simulink model "modello_completo_simulink2019"  (R2019b)
settings: Solver=VariableStepAuto  StartTime=0.0  StopTime=10  RelTol=1e-3
values from neighbouring files (symbols this model uses):
  a = 0.35    [data.m]    (also in geodetic2nedS.m = 6378137)
  a1 = rho * D^4 * alpha1    (= 0.000388302366464)    [data.m]
  a2 = -rho * D^3 * alpha2 * (1 - omega)    (= 0.0037030698432)    [data.m]
  AHRS_bias = [0 0 0]    [data.m]
  AHRS_sample_time = 1/50    (= 0.02)    [data.m]
  AHRS_var = ([1 1 2] * pi/180).^2    [data.m]
  alpha1 = 0.0113    [data.m]
  alpha2 = -0.0091    [data.m]
  c = son2(1)    [Sonar_id.m]    (also in data.m = 0.19)
  current = [seaCurrent; 0; 0; 0]    [data.m]
  D = 0.076    [data.m]
  dead_zone_limit = 31.5    [data.m]
  DVL_sample_t = 1/12    (= 0.0833333333333)    [data.m]
  DVL_var1 = 0.005^2    (= 2.5e-05)    [data.m]
  DVL_var2 = 0.015^2    (= 0.000225)    [data.m]
  DVL_var3 = 0.023^2    (= 0.000529)    [data.m]
  gps_sample_t = 1    [data.m]
  H = eye(3)    [data.m]    (also in navigation_data.m)
  IMU_sample_time = 1/100    (= 0.01)    [data.m]
  initial = []    [data.m]
  INSP = unicode2native(inspectionDirection)    [data.m]
  Ki_bodypos1 = 0    [parametri_PID.m]
  Ki_bodypos2 = 0    [parametri_PID.m]
  Ki_bodypos3 = 0    [parametri_PID.m]
  Ki_bodypos4 = 0    [parametri_PID.m]
  Ki_bodypos5 = 0    [parametri_PID.m]
  Ki_depth1 = 0    [parametri_PID.m]
  Ki_depth2 = 0    [parametri_PID.m]
  Ki_depth3 = 0    [parametri_PID.m]
  Ki_depth4 = 0    [parametri_PID.m]
  Ki_depth5 = 0    [parametri_PID.m]
  Ki_latvel1 = 0    [parametri_PID.m]
  Ki_latvel2 = 0    [parametri_PID.m]
  Ki_latvel3 = 0    [parametri_PID.m]
  Ki_latvel4 = 0    [parametri_PID.m]
  Ki_latvel5 = 0    [parametri_PID.m]
  Ki_P1 = 0    [parametri_PID.m]
  Ki_P2 = 0    [parametri_PID.m]
  Ki_P3 = 0    [parametri_PID.m]
  Ki_P4 = 0    [parametri_PID.m]
  Ki_P5 = 0    [parametri_PID.m]
  Ki_R1 = 0    [parametri_PID.m]
  Ki_R2 = 0    [parametri_PID.m]
  Ki_R3 = 0    [parametri_PID.m]
  Ki_R4 = 0    [parametri_PID.m]
  Ki_R5 = 0    [parametri_PID.m]
  Ki_rel_or1 = 0    [parametri_PID.m]
  Ki_rel_or2 = 0    [parametri_PID.m]
  Ki_rel_or3 = 0    [parametri_PID.m]
  Ki_rel_or4 = 0    [parametri_PID.m]
  Ki_rel_or5 = 0    [parametri_PID.m]
  Ki_reldist1 = 0    [parametri_PID.m]
  Ki_reldist2 = 0    [parametri_PID.m]
  Ki_reldist3 = 0    [parametri_PID.m]
  Ki_reldist4 = 0    [parametri_PID.m]
  Ki_reldist5 = 0    [parametri_PID.m]
  Ki_surge1 = 0    [parametri_PID.m]
  Ki_surge2 = 0    [parametri_PID.m]
  Ki_surge3 = 0    [parametri_PID.m]
  Ki_surge4 = 0    [parametri_PID.m]
  Ki_surge5 = 0    [parametri_PID.m]
  Ki_yaw1 = 0    [parametri_PID.m]
  Ki_yaw2 = 0    [parametri_PID.m]
  Ki_yaw3 = 0    [parametri_PID.m]
  Ki_yaw4 = 0    [parametri_PID.m]
  Ki_yaw5 = 0    [parametri_PID.m]
  Kp_bodypos1 = 0    [parametri_PID.m]
  Kp_bodypos2 = 2    [parametri_PID.m]
  Kp_bodypos3 = 2    [parametri_PID.m]
  Kp_bodypos4 = 2    [parametri_PID.m]
  Kp_bodypos5 = 2    [parametri_PID.m]
  Kp_depth1 = 0    [parametri_PID.m]
  Kp_depth2 = 2    [parametri_PID.m]
  Kp_depth3 = 2    [parametri_PID.m]
  Kp_depth4 = 2    [parametri_PID.m]
  Kp_depth5 = 2    [parametri_PID.m]
  Kp_latvel1 = 0    [parametri_PID.m]
  Kp_latvel2 = 2    [parametri_PID.m]
  Kp_latvel3 = 2    [parametri_PID.m]
  Kp_latvel4 = 2    [parametri_PID.m]
  Kp_latvel5 = 2    [parametri_PID.m]
  Kp_P1 = 0    [parametri_PID.m]
  Kp_P2 = 2    [parametri_PID.m]
  Kp_P3 = 2    [parametri_PID.m]
  Kp_P4 = 2    [parametri_PID.m]
  Kp_P5 = 2    [parametri_PID.m]
  Kp_R1 = 0    [parametri_PID.m]
  Kp_R2 = 2    [parametri_PID.m]
  Kp_R3 = 2    [parametri_PID.m]
  Kp_R4 = 2    [parametri_PID.m]
  Kp_R5 = 2    [parametri_PID.m]
  Kp_rel_or1 = 0    [parametri_PID.m]
  Kp_rel_or2 = 2    [parametri_PID.m]
  Kp_rel_or3 = 2    [parametri_PID.m]
  Kp_rel_or4 = 2    [parametri_PID.m]
  Kp_rel_or5 = 2    [parametri_PID.m]
  Kp_reldist1 = 0    [parametri_PID.m]
  Kp_reldist2 = 2    [parametri_PID.m]
  Kp_reldist3 = 2    [parametri_PID.m]
  Kp_reldist4 = 2    [parametri_PID.m]
  Kp_reldist5 = 2    [parametri_PID.m]
  Kp_surge1 = 0    [parametri_PID.m]
  Kp_surge2 = 2    [parametri_PID.m]
  Kp_surge3 = 2    [parametri_PID.m]
  Kp_surge4 = 2    [parametri_PID.m]
  Kp_surge5 = 2    [parametri_PID.m]
  Kp_yaw1 = 0.6*6    (= 3.6)    [parametri_PID.m]
  Kp_yaw2 = 2    [parametri_PID.m]
  Kp_yaw3 = 2    [parametri_PID.m]
  Kp_yaw4 = 2    [parametri_PID.m]
  Kp_yaw5 = 2    [parametri_PID.m]
  M = M_rb + M_a    [Masse.m]
  M_inv = inv(M)    [Masse.m]
  n_max = 340    [data.m]
  num_cycle = 5    [data.m]    (also in navigation_data.m)
  omega = 0.1    [data.m]
  plot_smpl = 0.1    [data.m]
  ps_sample_t = 0.02    [data.m]
  ps_var = (5000/3)^2    (= 2777777.77778)    [data.m]
  pylonCenter = [ 43.723046 ... (first row only)    [missionB.m]
  ... (+4 more)
undefined symbols (not defined in the file or in its folder): DiscIntNeverNeededParam, s_data
libraries: simulink x3
(part 5 of 6)

== system modello_completo_simulink2019/Vehicle Model/Thrusters/T/Thruster 4 ==
  note: n is the rotational speed of the thruster
      | V is the speed component of the water along the thruster axis
      |
      | n is saturated according to data
      | a dead zone is considered according to data
      | the thruster is characterised by 1st order dynamics (tau = 0.2s)
  n [rad/s] : Inport
  V [m/s] : Inport  Port=2
  Dead Zone : DeadZone  LowerValue=-dead_zone_limit  UpperValue=dead_zone_limit  SaturateOnIntegerOverflow=on
  MATLAB Function : MATLAB Function  TreatAsAtomicUnit=on
  Saturation : Saturate  UpperLimit=n_max  LowerLimit=-n_max
  Transfer Fcn : TransferFcn  Denominator=[0.2 1]
  T i : Outport
  wires:
  V [m/s]/1 -> MATLAB Function/2(V)
  Saturation/1 -> MATLAB Function/1(n)
  Transfer Fcn/1 -> Saturation/1
  Dead Zone/1 -> Transfer Fcn/1
  n [rad/s]/1 -> Dead Zone/1
  MATLAB Function/1(T) -> T i/1

== system modello_completo_simulink2019/Vehicle Model/Thrusters/T/Thruster 5 ==
  note: n is the rotational speed of the thruster
      | V is the speed component of the water along the thruster axis
      |
      | n is saturated according to data
      | a dead zone is considered according to data
      | the thruster is characterised by 1st order dynamics (tau = 0.2s)
  n [rad/s] : Inport
  V [m/s] : Inport  Port=2
  Dead Zone : DeadZone  LowerValue=-dead_zone_limit  UpperValue=dead_zone_limit  SaturateOnIntegerOverflow=on
  MATLAB Function : MATLAB Function  TreatAsAtomicUnit=on
  Saturation : Saturate  UpperLimit=n_max  LowerLimit=-n_max
  Transfer Fcn : TransferFcn  Denominator=[0.2 1]
  T i : Outport
  wires:
  V [m/s]/1 -> MATLAB Function/2(V)
  Saturation/1 -> MATLAB Function/1(n)
  Transfer Fcn/1 -> Saturation/1
  Dead Zone/1 -> Transfer Fcn/1
  n [rad/s]/1 -> Dead Zone/1
  MATLAB Function/1(T) -> T i/1

== system modello_completo_simulink2019/Vehicle Model/Thrusters/T/Thruster 6 ==
  note: n is the rotational speed of the thruster
      | V is the speed component of the water along the thruster axis
      |
      | n is saturated according to data
      | a dead zone is considered according to data
      | the thruster is characterised by 1st order dynamics (tau = 0.2s)
  n [rad/s] : Inport
  V [m/s] : Inport  Port=2
  Dead Zone : DeadZone  LowerValue=-dead_zone_limit  UpperValue=dead_zone_limit  SaturateOnIntegerOverflow=on
  MATLAB Function : MATLAB Function  TreatAsAtomicUnit=on
  Saturation : Saturate  UpperLimit=n_max  LowerLimit=-n_max
  Transfer Fcn : TransferFcn  Denominator=[0.2 1]
  T i : Outport
  wires:
  V [m/s]/1 -> MATLAB Function/2(V)
  Saturation/1 -> MATLAB Function/1(n)
  Transfer Fcn/1 -> Saturation/1
  Dead Zone/1 -> Transfer Fcn/1
  n [rad/s]/1 -> Dead Zone/1
  MATLAB Function/1(T) -> T i/1

== system modello_completo_simulink2019/Vehicle Model/Thrusters/T/Thruster 7 ==
  note: n is the rotational speed of the thruster
      | V is the speed component of the water along the thruster axis
      |
      | n is saturated according to data
      | a dead zone is considered according to data
      | the thruster is characterised by 1st order dynamics (tau = 0.2s)
  n [rad/s] : Inport
  V [m/s] : Inport  Port=2
  Dead Zone : DeadZone  LowerValue=-dead_zone_limit  UpperValue=dead_zone_limit  SaturateOnIntegerOverflow=on
  MATLAB Function : MATLAB Function  TreatAsAtomicUnit=on
  Saturation : Saturate  UpperLimit=n_max  LowerLimit=-n_max
  Transfer Fcn : TransferFcn  Denominator=[0.2 1]
  T i : Outport
  wires:
  V [m/s]/1 -> MATLAB Function/2(V)
  Saturation/1 -> MATLAB Function/1(n)
  Transfer Fcn/1 -> Saturation/1
  Dead Zone/1 -> Transfer Fcn/1
  n [rad/s]/1 -> Dead Zone/1
  MATLAB Function/1(T) -> T i/1

== matlab function modello_completo_simulink2019/Vehicle Model/Model Vehicle/D ==
  data: ni_r input; F_d output; rho input
function F_d = D_forces(ni_r, rho)
    % Funzione per il calcolo delle forze di drag (Formulazione tratta da
    % Fossen(2011))
    %
    % IN: ni_r [6x1] | velocità lineare [3x1] m/s, velocità angolare [3x1] rad/s 
    %                  differenza tra velocità del centro di massa del
    %                  veicolo in terna NED e velocità della corrente
    %     rho  [1x1] | densità dell'acqua kg/m^3
    %
    % OUT: F_d [6x1] | forze [3x1] N, momenti [3x1] N*m dovuti a effetti di
    %                  drag
    %
    
    ni_lin = ni_r(1:3); 
    ni_ang = ni_r(4:6);
    
    % semiassi del veicolo
    a = 0.35; 
    b = a;
    c = 0.19;
    
    A_ab = pi*a*b;      % Area su cui agisce la forza di drag lin lungo z, momento di drag intorno a x e y
    A_bc = pi*b*c;      % Area su cui agisce la forza di drag lin lungo x, momento di drag intorno a z
    A_ac = pi*a*c;      % Area su cui agisce la forza di drag lin lungo y

    Di = 0.7; % diametro m massimo del veicolo, supposto il veicolo una sfera
    
    % Calcolo del numero di Reynolds basato su una velocità operativa di
    % 0.3 m/s, viscosità del fluido di 1e-3 Pa*s, calcolata a una
    % temperatura di 20 °C e con una densità di 1030 kg/m^3
    visc = 1e-3;
    vmax = 3e-1;
    rho  = 1030;
    Re = Di/(visc/rho)*vmax; % Re = 2*1e5
 
    Cd = 0.49; % Coefficiente di drag ricavato da Re nel caso di una sfera liscia
    
    % Calcolo dei raggi medi delle semiellisse di applicazione del momento
    % di drag
    
    rm_z = 4*c/(3*pi);
    rm_xy = 4*a/(3*pi);
    
    D_lin = -1/2*rho*Cd*diag([A_bc, A_ac, A_ab])*(abs(ni_lin).*ni_lin); % Forze lineari
    D_ang = -1/2*rho*Cd*diag([rm_xy^3*A_ab, rm_xy^3*A_ab, rm_z^3*A_bc])*(abs(ni_ang).*ni_ang); % Momenti
    
    F_d = [D_lin; D_ang];
end

== matlab function modello_completo_simulink2019/Vehicle Model/Model Vehicle/C ==
  data: ni_r input; F_c output; M input
function F_c = C(ni_r, M)
    % Funzione per il calcolo delle forze e dei momenti di Coriolis e
    % centripete (Formulazione tratta dal Fossen(2011))
    
    % IN: ni_r [6x1] | velocità lineare [3x1] m/s, velocità angolare [3x1] rad/s 
    %                  differenza tra velocità del centro di massa del
    %                  veicolo in terna NED e velocità della corrente
    %     M    [6x6] | matrice delle masse
    
    % OUT: F_c [6x1] | forze [3x1] N, momenti [3x1] N*m dovuti a effetti di
    %                  Coriolis e accelerazione centripeta
    
    ni = ni_r;
    M11 = M(1:3,1:3);
    M22 = M(4:6,4:6);
    ni1 = ni(1:3);
    ni2 = ni(4:6);
    C11 = zeros(3,3);
    s1 = M11*ni1;
    C12 = - [0 -s1(3) s1(2); s1(3) 0 -s1(1); -s1(2) s1(1) 0];
    C21 = C12;
    s2 = M22*ni2;
    C22 = - [0 -s2(3) s2(2); s2(3) 0 -s2(1); -s2(2) s2(1) 0];
    F_c = [C11 C12; C21 C22]*ni_r;
end

== matlab function modello_completo_simulink2019/Vehicle Model/Model Vehicle/grav ==
  data: rho input; eta input; F_g output
function F_g = grav(rho, eta)
    % Funzione per il calcolo delle forze di gravità e galleggiamento del
    % veicolo (Formulazione tratta da Fossen(2011))
    %
    % IN: rho  [1x1] | densità dell'acqua kg/m^3
    %     eta  [6x1] | posizione [3x1] m, orientazione [3x1] rad del veicolo in terna NED
    %
    % OUT: F_g [6x1] | forze [3x1] N, momenti [3x1] N*m dovuti a effetti di
    %                  gravità e galleggiamento
    %
    
    eta2 = eta(4:6);
    g = 9.81; % m/s^2 modulo della accelerazione di gravità
    
    % semiassi m del veicolo
    a = 0.35;
    b = a;
    c = 0.19;
    
    massa = 100; % massa kg del veicolo
    
    % Calcolo della calotta dell'ellissoide emersa dall'acqua per simulare 
    % il comportamento del veicolo emerso 
    
    if eta(3) >= c
       V = 4/3*pi*a*b*c; % volume del veicolo totalmente immerso
    else
       V = 4/3*pi*a*b*c - (pi*a*b/(3*c^2))*((eta(3)-c)^2)*(3*c - abs(eta(3) - c)); % volume del veicolo parzialmente immerso
    end
    
    
    W = massa*g; % modulo forza di gravità
    B = rho*V*g; % modulo forza di galleggiamento
    
    % Passaggio da terna NED a Body
    J = Jac(eta2);
    J1 = J(1:3,1:3);
    J2 = J(4:6,4:6);
    
    f_g = inv(J1)*[0; 0; W];
    f_b = inv(J1)*[0; 0; -B];
    r_g = [0; 0; 0]; % posizione del centro di massa
    r_b = [0; 0; -c/2]; % posizione del centro di galleggiamento

    F_g = -[f_g + f_b; cross(r_g,f_g) + cross(r_b,f_b)];
end

== matlab function modello_completo_simulink2019/Vehicle Model/Model Vehicle/Kinematic/Jac ==
  data: eta input; J output
function J = Jac(eta)
    % Funzione per il calcolo dello Jacobiano per il passaggio da
    % coordinate Body a coordinate NED
    %
    % IN: eta2 [3x1] rad angoli di roll, pitch, yaw
    %
    % OUT: J [6x6] Jacobiano complessivo
    %
    eta2 = eta(4:6);
    phi = eta2(1);
    theta = eta2(2);
    psi = eta2(3);
    Rx = [1 0 0; 0 cos(phi) sin(phi); 0 -sin(phi) cos(phi)]; % Rot elementare attorno a x
    Ry = [cos(theta) 0 -sin(theta); 0 1 0; sin(theta) 0 cos(theta)]; % Rot elementare attorno a y
    Rz = [cos(psi) sin(psi) 0; -sin(psi) cos(psi) 0; 0 0 1]; % Rot elementare attorno a z
    J1 = Rz'*Ry'*Rx'; % Jacobiano per il passaggio da Body a NED delle componenti lineari
    J2 = [1 sin(phi)*tan(theta) cos(phi)*tan(theta); ... % Jacobiano per il passaggio da Body a NED delle componenti angolari
        0 cos(phi) -sin(phi); ...
        0 sin(phi)/cos(theta) cos(phi)/cos(theta)];
    J = blkdiag(J1, J2);
end

== matlab function modello_completo_simulink2019/Vehicle Model/Thrusters/T/Thruster 1/MATLAB Function ==
  data: n input; T output; V input; D parameter; omega parameter; a1 parameter; a2 parameter; alpha1 parameter; alpha2 parameter
function T = thrusterModel(n, V, D, omega, a1, a2, alpha1, alpha2)

Va = (1-omega) * V;     % Advancement velocity at the propeller
J0 = Va/(n*D);          % Advancement Coefficient

if J0 > -alpha1/alpha2  % Out of linearity domain (right side)
    T = 0;              % A null generated thrust is assumed
    
elseif J0 < 0           % Out of linearity domain (left side)
    T = a1*abs(n)*n;    % Bollard thrust is assumed

else                    % Within the linearity domain
    T = a1*abs(n)*n - a2*abs(n)*V;
end

== matlab function modello_completo_simulink2019/Vehicle Model/Thrusters/T/Thruster 2/MATLAB Function ==
  data: n input; T output; V input; D parameter; omega parameter; a1 parameter; a2 parameter; alpha1 parameter; alpha2 parameter
function T = thrusterModel(n, V, D, omega, a1, a2, alpha1, alpha2)

Va = (1-omega) * V;     % Advancement velocity at the propeller
J0 = Va/(n*D);          % Advancement Coefficient

if J0 > -alpha1/alpha2  % Out of linearity domain (right side)
    T = 0;              % A null generated thrust is assumed
    
elseif J0 < 0           % Out of linearity domain (left side)
    T = a1*abs(n)*n;    % Bollard thrust is assumed

else                    % Within the linearity domain
    T = a1*abs(n)*n - a2*abs(n)*V;
end

== matlab function modello_completo_simulink2019/Vehicle Model/Thrusters/T/Thruster 3/MATLAB Function ==
  data: n input; T output; V input; D parameter; omega parameter; a1 parameter; a2 parameter; alpha1 parameter; alpha2 parameter
function T = thrusterModel(n, V, D, omega, a1, a2, alpha1, alpha2)

Va = (1-omega) * V;     % Advancement velocity at the propeller
J0 = Va/(n*D);          % Advancement Coefficient

if J0 > -alpha1/alpha2  % Out of linearity domain (right side)
    T = 0;              % A null generated thrust is assumed
    
elseif J0 < 0           % Out of linearity domain (left side)
    T = a1*abs(n)*n;    % Bollard thrust is assumed

else                    % Within the linearity domain
    T = a1*abs(n)*n - a2*abs(n)*V;
end

== matlab function modello_completo_simulink2019/Vehicle Model/Thrusters/T/Thruster 4/MATLAB Function ==
  data: n input; T output; V input; D parameter; omega parameter; a1 parameter; a2 parameter; alpha1 parameter; alpha2 parameter
function T = thrusterModel(n, V, D, omega, a1, a2, alpha1, alpha2)

Va = (1-omega) * V;     % Advancement velocity at the propeller
J0 = Va/(n*D);          % Advancement Coefficient

if J0 > -alpha1/alpha2  % Out of linearity domain (right side)
    T = 0;              % A null generated thrust is assumed
    
elseif J0 < 0           % Out of linearity domain (left side)
    T = a1*abs(n)*n;    % Bollard thrust is assumed

else                    % Within the linearity domain
    T = a1*abs(n)*n - a2*abs(n)*V;
end

== matlab function modello_completo_simulink2019/Vehicle Model/Thrusters/T/Thruster 5/MATLAB Function ==
  data: n input; T output; V input; D parameter; omega parameter; a1 parameter; a2 parameter; alpha1 parameter; alpha2 parameter
function T = thrusterModel(n, V, D, omega, a1, a2, alpha1, alpha2)

Va = (1-omega) * V;     % Advancement velocity at the propeller
J0 = Va/(n*D);          % Advancement Coefficient

if J0 > -alpha1/alpha2  % Out of linearity domain (right side)
    T = 0;              % A null generated thrust is assumed
    
elseif J0 < 0           % Out of linearity domain (left side)
    T = a1*abs(n)*n;    % Bollard thrust is assumed

else                    % Within the linearity domain
    T = a1*abs(n)*n - a2*abs(n)*V;
end

== matlab function modello_completo_simulink2019/Vehicle Model/Thrusters/T/Thruster 6/MATLAB Function ==
  data: n input; T output; V input; D parameter; omega parameter; a1 parameter; a2 parameter; alpha1 parameter; alpha2 parameter
function T = thrusterModel(n, V, D, omega, a1, a2, alpha1, alpha2)

Va = (1-omega) * V;     % Advancement velocity at the propeller
J0 = Va/(n*D);          % Advancement Coefficient

if J0 > -alpha1/alpha2  % Out of linearity domain (right side)
    T = 0;              % A null generated thrust is assumed
    
elseif J0 < 0           % Out of linearity domain (left side)
    T = a1*abs(n)*n;    % Bollard thrust is assumed

else                    % Within the linearity domain
    T = a1*abs(n)*n - a2*abs(n)*V;
end

== matlab function modello_completo_simulink2019/Vehicle Model/Thrusters/T/Thruster 7/MATLAB Function ==
  data: n input; T output; V input; D parameter; omega parameter; a1 parameter; a2 parameter; alpha1 parameter; alpha2 parameter
function T = thrusterModel(n, V, D, omega, a1, a2, alpha1, alpha2)

Va = (1-omega) * V;     % Advancement velocity at the propeller
J0 = Va/(n*D);          % Advancement Coefficient

if J0 > -alpha1/alpha2  % Out of linearity domain (right side)
    T = 0;              % A null generated thrust is assumed
    
elseif J0 < 0           % Out of linearity domain (left side)
    T = a1*abs(n)*n;    % Bollard thrust is assumed

else                    % Within the linearity domain
    T = a1*abs(n)*n - a2*abs(n)*V;
end

== matlab function modello_completo_simulink2019/Vehicle Model/Model Vehicle/MATLAB Function ==
  data: coord_pylon input; eta input; eta_ecef output
function eta_ecef = nedToEcef(coord_pylon, eta) 
    % Funzione per il passaggio da coordinate in terna NED a coordinate in
    % terna geodetica.
    %
    % IN: coord_pylon [3x1] | latitudine e longitudine [2x1] deg,
    %                         profondità [1x1] m
    %     eta         [6x1] | posizione [3x1] m, orientazione [3x1] rad 
    %                         del veicolo in terna NED
    
    % OUT: eta_ecef   [6x1] | posizione [3x1] m, orientazione [3x1] rad 
    %                         del veicolo in terna ecef
    
    coder.extrinsic('wgs84Ellipsoid');

    coder.extrinsic('ned2geodetic');
    
    eta_pos = eta(1:6);
    wgs84 = wgs84Ellipsoid('meter'); 
    [eta_pos(1), eta_pos(2)] = ned2geodetic(eta(1), eta(2), eta(3), coord_pylon(1), coord_pylon(2), coord_pylon(3), wgs84, 'degrees');
    
    eta_pos(3) = eta(3);
    eta_pos(4:6) = eta_pos(4:6);
    
    eta_ecef = eta_pos;
    
end

== matlab function modello_completo_simulink2019/Vehicle Model/MATLAB Function ==
  data: eta input; ni_c output; current input
function ni_c = current_ned2body(eta, current)
    % Funzione per il calcolo della velocità della corrente in terna Body
    
    % IN: eta     [6x1] | posizione [3x1] m, orientazione [3x1] rad del veicolo in terna NED
    %     current [6x1] | velocità lineare [3x1] m/s, velocità angolare
    %                     [3x1] rad/s (sempre nulla) della corrente in
    %                     terna NED


    % OUT: ni_c   [6x1] | velocità lineare [3x1] m/s, velocità angolare
    %                     [3x1] rad/s (sempre nulla) della corrente in
    %                     terna Body
    
    eta2 = eta(4:6);            % eta2 espresso in radianti
    ni_c = Jac(eta2)'*current;
end

== matlab function modello_completo_simulink2019/Vehicle Model/Thrusters/T/MATLAB Function ==
  data: ni_r input; v_th output
function v_th = thrusters(ni_r) 
    % Funzione per valutare le componenti di velocità di ciascun thruster
    % in direzione del proprio asse 
    
    % IN: ni_r [6x1] | velocità lineare [3x1] m/s, velocità angolare [3x1] rad/s 
    %                  differenza tra velocità del centro di massa del
    %                  veicolo in terna NED e velocità della corrente

    
    % OUT: v_th [7x1] m/s componenti di velocità relativa lungo l'asse di
    % ciascun thruster
    
    % posizionamento dei thrusters
    p1 = [0 -0.25 0]';
    p2 = [0 0.25 0]';
    p3 = [-0.25 0 0]';
    p4 = [0.25 0 0]';
    p5 = [-0.15 -0.15 0]';
    p6 = [-0.15 0.15 0]';
    p7 = [0.15 0 0]';


    % versori posizionamento dei thrusters
    t1 = [1 0 0]';
    t2 = t1;
    t3 = [0 1 0]';
    t4 = -t3;
    t5 = [0 0 1]';
    t6 = t5;
    t7 = t5;

    v_lin = ni_r(1:3); % componenti di velocità lineare
    v_ang = ni_r(4:6); % componenti di velocità angolare

    % velocità lineari dei punti p_i (centro dei thrusters) attraverso la formula
    % fondamentale della cinematica
    vp1 = v_lin + cross(v_ang, p1); 
    vp2 = v_lin + cross(v_ang, p2);
    vp3 = v_lin + cross(v_ang, p3);
    vp4 = v_lin + cross(v_ang, p4);
    vp5 = v_lin + cross(v_ang, p5);
    vp6 = v_lin + cross(v_ang, p6);
    vp7 = v_lin + cross(v_ang, p7);

    % velocità relativa lungo l'asse di ciascun thruster 
    v1 = vp1'*t1;
    v2 = vp2'*t2;
    v3 = vp3'*t3;
    v4 = vp4'*t4;
    v5 = vp5'*t5;
    v6 = vp6'*t6;
    v7 = vp7'*t7;

    v_th = [ v1 v2 v3 v4 v5 v6 v7]'; % OUT
end

== matlab function modello_completo_simulink2019/Navigation1/Geodetic to NED/MATLAB Function2 ==
  data: GPS_geodetic input; GPS_flag input; GPS_NED output; depth input; pylonCenter parameter
function GPS_NED = Geo2NED(GPS_geodetic, GPS_flag, depth, pylonCenter)

% Funzione che trasforma le coordinate dal sistema di riferimento geodetico
% ad un sistema NED con origine in corrispondenza del centro del pilone.

%% GPS non funzionante
if GPS_flag == 0            
    GPS_NED = [0;0;0];
    return
end

%% Variabili
phi = GPS_geodetic(1);                  % Coordinate geodetiche in radianti                     
lambda = GPS_geodetic(2);  
h = -depth;

phi_pyl = pylonCenter(1) * pi/180;      % Origine del sistema NED in coordinate geodetiche
lambda_pyl = pylonCenter(2) * pi/180;

%% Trasformazione coordinate
coder.extrinsic('wgs84Ellipsoid');
coder.extrinsic('geodetic2ned');
    
[x_gps2, y_gps2, z_gps2] = geodetic2ned(phi, lambda, -depth, phi_pyl, lambda_pyl, 0, wgs84Ellipsoid, 'radians');
eta_NED_GPS = [x_gps2; y_gps2];

GPS_NED = zeros(3,1);
GPS_NED(1) = eta_NED_GPS(1);            % Coordiante NED in radianti
GPS_NED(2) = eta_NED_GPS(2);
GPS_NED(3) = GPS_flag;

== matlab function modello_completo_simulink2019/Vehicle Model/Thrusters/saturation_tau ==
  data: tau input; tau_sat output; eta input
function tau_sat = sat_tau(tau, eta)
    % Funzione per la saturazione della spinta verso l'alto in uscita al blocco 
    % dei thrusters nell'ipotesi in cui il veicolo si trovi in superficie
    % con angoli di yaw, pitch e roll supposti piccoli a piacere

    % IN: tau [6x1] | forze [3x1] N, momenti [3x1] N*m agenti sul veicolo
    %     eta [6x1] | posizione [3x1] m, orientazione [3x1] rad del veicolo in terna NED
    
    % OUT: tau_sat [6x1] | forze saturate [3x1] N e momenti [3x1] N*m agenti sul veicolo
    
    tau_sat = [0;0;0;0;0;0];
    tau_sat = tau;

    if eta(3) < 0.1 % condizione per il veicolo in superficie
        tau_sat(3) = 0;
    end
    
end

== matlab function modello_completo_simulink2019/Vehicle Model/MATLAB Function1 ==
  data: Tdes input; n output
function n  = fcn(Tdes)
n=zeros(1,7)';
a1=0.000388302366464000;
%assunzione modello a bassa velocità
for i=1:1:7
       n(i)=sign(Tdes(i))*sqrt((abs(Tdes(i))/a1));  
end
end

== matlab function modello_completo_simulink2019/Navigation1/MATLAB Function1 ==
  data: ang_vel input; DVL input; nu_1 output; c parameter
function nu_1  = dvl2body(ang_vel, DVL, c)

% Funzione che si occupa di trasformare la velocità da sistema di
% riferimento associato al DVL al sistema BODY

% nu_dvl = R_b^dvl (nu_1 + S(nu_2)* P_dvl)
% nu_1 = R_b^dvl' * nu_dvl - S(nu_2) * P_dvl

nu_1    =   zeros(4,1);
nu_2    =   [ang_vel(1); ang_vel(2); ang_vel(3)];
vel_dvl =   [DVL(1); DVL(2); DVL(3)];
R_b_dvl =   eye(3);

S = [   0,          -nu_2(3),   nu_2(2); 
        nu_2(3),    0,          -nu_2(1); 
        -nu_2(2),   nu_2(1),    0       ];
    
p = [0;0;c];

nu_1(1:3) = R_b_dvl' * vel_dvl - S * p;
nu_1(4) = DVL(4); %Flag

== matlab function modello_completo_simulink2019/Navigation1/MATLAB Function2 ==
  data: Depth_ps input; Depth output; c parameter
function  Depth = ps2body(Depth_ps, c)
% Il profondimetro è posizionato nella parte inferiore dell'AUV, lungo
% l'asse z
Depth = zeros(2,1);
Depth(1) = Depth_ps(1) - c;     %profondità rispetto al centro di massa
Depth(2) = Depth_ps(2);         %flag

== matlab function modello_completo_simulink2019/Navigation1/AHRS_function ==
  data: eta2 output; lin_acc input; nu2 output; ang_vel input; orientation input
function [eta2, nu2]= AHRS_signals(lin_acc, ang_vel, orientation)
acc = lin_acc(1:3);
nu2 = ang_vel(1:3);
eta2 = orientation(1:3);

== matlab function modello_completo_simulink2019/Navigation1/DVL_function ==
  data: dvl input; velocity_est output; flag_DVL output
function [velocity_est, flag_DVL] = DVL_signals(dvl)
velocity_est = dvl(1:3);
flag_DVL = dvl(4);

== matlab function modello_completo_simulink2019/Navigation1/NED to Geodetic/MATLAB Function1 ==
  data: eta_NED input; eta_geodetic output; depth input; pylonCenter parameter
function eta_geodetic = NED2Geo(eta_NED, depth, pylonCenter)

% Funzione che trasforma le coordinate dal sistema NED con origine in
% corrispondenza del centro del pilone al sistema di riferimento geodetico

phi_pyl = pylonCenter(1) * pi/180;      % Origine del sistema NED in coordinate geodetiche 
lambda_pyl = pylonCenter(2) * pi/180;

%% Trasformazione
coder.extrinsic('wgs84Ellipsoid');
coder.extrinsic('ned2geodetic');

[lat, lon, h] = ned2geodetic(eta_NED(1), eta_NED(2), depth, phi_pyl, lambda_pyl, 0, wgs84Ellipsoid, 'radians');

eta_geodetic = [0; 0];
eta_geodetic = [lat; lon];              % Coordiante geodetiche in radianti

== matlab function modello_completo_simulink2019/Navigation1/Relative estimation/Sonar trigger/MATLAB Function ==
  data: sonar input; sum input; pulse output; prev output
function [pulse, prev] = fcn(sonar, sum)

% La funzione si occupa di monitorare la misura dei sonar,
% quando esse sono modificate manda un impulso al blocco di stima relativa

if nnz(isnan(sum)) > 0 || nnz(sum) == 0 
    pulse = 0;
else
    pulse = 1;
end

prev = sonar;

== matlab function modello_completo_simulink2019/Navigation1/Relative estimation/Subsystem/MATLAB Function9 ==
  data: sonar input; orientation input; distance output; alpha output; flag_sonar output; pylonRadius parameter; a parameter; s_data parameter
function [distance, alpha, flag_sonar] = relative_values(sonar, orientation, pylonRadius, a, s_data)

% Chiamando la funzione "fcn_sonar" si occupa di calcolate la distanza
% e l'angolo dell'AUV rispetto al pilone

distance = 0;
alpha = 0;
flag_sonar = 0;

coder.extrinsic('fcn_sonar');

[distance, alpha, flag_sonar] = fcn_sonar(sonar, orientation, pylonRadius, a, s_data);
end

== matlab function modello_completo_simulink2019/Navigation1/flag_function ==
  data: flag_depth input; flag_AHRS input; error_flag output; flag_DVL input; flag_sonar input
function error_flag = fcn(flag_depth, flag_AHRS, flag_DVL, flag_sonar)

% Funzione che rileva la presenza di errore in un sensore

flag_ahrs = flag_AHRS(1) & flag_AHRS(2) & flag_AHRS(3);
error_flag = ~(flag_depth & flag_ahrs & flag_DVL & flag_sonar); % Vale 1 se vi è un errore

== matlab function modello_completo_simulink2019/Navigation1/z_EKF/EXTENDED KALMAN FILTER/Correzione  ==
  data: prev_pos output; prev_pos input; P input; hat input; meas_pos input; GPS_flag input; meas_depth input; P output; hat output; R parameter; H parameter
function [prev_pos, P, hat] = EKF_pos(prev_pos, P, hat, meas_pos, GPS_flag, meas_depth, R, H)
%% EKF: Correction

% Il filtro corregge i valori di posizione x e y solo quando è disponibile una nuova misura del GPS
if nnz(round(10.^4*(meas_pos - prev_pos))/10.^4) ~= 0 && GPS_flag == 1       % Se il flag è 0 il GPS non funziona

    z_tilde = [ meas_pos(1) - hat(1);
                meas_pos(2) - hat(2);
                meas_depth - hat(3)];

else
        z_tilde = [ 0;
                    0;
                meas_depth - hat(3)];
end
            
    S = H * P * H' + R;

    K = P * H' * S^(-1);
    
    hat = hat + K * z_tilde;
    P = (eye(3) - K * H) * P;  

prev_pos = meas_pos;

== matlab function modello_completo_simulink2019/Navigation1/z_EKF/EXTENDED KALMAN FILTER/Predizione ==
  data: P input; hat input; dT input; P output; hat output; orientation input; dvl input; ahrs_flag input; init input; P0 input; Q parameter
function [P, hat]  = EKF_pos(P, hat, dT, orientation, dvl, ahrs_flag, init, P0, Q)

dvl_flag = dvl(4);

%% Inizializzazione stato e matrice P
if nnz(hat) == 0           
    hat= init;
    P = P0;
end

if (ahrs_flag && dvl_flag) == 1
    %% Calcolo variabili e matrici
    phi     =   orientation(1);             % roll
    theta   =   orientation(2);             % pitch
    psi_    =   orientation(3);             % yaw
    vel     =   [dvl(1); dvl(2); dvl(3)];  
    
    J       =   zeros(3,3);
    Lk      =   zeros(3,6);
    
    J = [ cos(psi_)*cos(theta), cos(psi_)*sin(phi)*sin(theta) - cos(phi)*sin(psi_), sin(phi)*sin(psi_) + cos(phi)*cos(psi_)*sin(theta);
       cos(theta)*sin(psi_), cos(phi)*cos(psi_) + sin(phi)*sin(psi_)*sin(theta), cos(phi)*sin(psi_)*sin(theta) - cos(psi_)*sin(phi);
         -sin(theta),                                cos(theta)*sin(phi),                                cos(phi)*cos(theta)];
     
    x = dvl(1);
    y = dvl(2);
    z = dvl(3);
    n_ahrs1 = 0;
    n_ahrs2 = 0;
    n_ahrs3 = 0;

    % Matrice Lk: derivata della funzione f rispetto al rumore di AHRS e
    % DVL
    Lk = [  dT*(y*(sin(n_ahrs1 + phi)*sin(n_ahrs3 + psi_) + cos(n_ahrs1 + phi)*cos(n_ahrs3 + psi_)*sin(n_ahrs2 + theta)) + z*(cos(n_ahrs1 + phi)*sin(n_ahrs3 + psi_) - cos(n_ahrs3 + psi_)*sin(n_ahrs1 + phi)*sin(n_ahrs2 + theta))), dT*(z*cos(n_ahrs1 + phi)*cos(n_ahrs3 + psi_)*cos(n_ahrs2 + theta) - x*cos(n_ahrs3 + psi_)*sin(n_ahrs2 + theta) + y*cos(n_ahrs3 + psi_)*cos(n_ahrs2 + theta)*sin(n_ahrs1 + phi)), -dT*(y*(cos(n_ahrs1 + phi)*cos(n_ahrs3 + psi_) + sin(n_ahrs1 + phi)*sin(n_ahrs3 + psi_)*sin(n_ahrs2 + theta)) - z*(cos(n_ahrs3 + psi_)*sin(n_ahrs1 + phi) - cos(n_ahrs1 + phi)*sin(n_ahrs3 + psi_)*sin(n_ahrs2 + theta)) + x*cos(n_ahrs2 + theta)*sin(n_ahrs3 + psi_)), dT*cos(n_ahrs3 + psi_)*cos(n_ahrs2 + theta), -dT*(cos(n_ahrs1 + phi)*sin(n_ahrs3 + psi_) - cos(n_ahrs3 + psi_)*sin(n_ahrs1 + phi)*sin(n_ahrs2 + theta)),  dT*(sin(n_ahrs1 + phi)*sin(n_ahrs3 + psi_) + cos(n_ahrs1 + phi)*cos(n_ahrs3 + psi_)*sin(n_ahrs2 + theta));
     -dT*(y*(cos(n_ahrs3 + psi_)*sin(n_ahrs1 + phi) - cos(n_ahrs1 + phi)*sin(n_ahrs3 + psi_)*sin(n_ahrs2 + theta)) + z*(cos(n_ahrs1 + phi)*cos(n_ahrs3 + psi_) + sin(n_ahrs1 + phi)*sin(n_ahrs3 + psi_)*sin(n_ahrs2 + theta))), dT*(z*cos(n_ahrs1 + phi)*cos(n_ahrs2 + theta)*sin(n_ahrs3 + psi_) - x*sin(n_ahrs3 + psi_)*sin(n_ahrs2 + theta) + y*cos(n_ahrs2 + theta)*sin(n_ahrs1 + phi)*sin(n_ahrs3 + psi_)),  dT*(z*(sin(n_ahrs1 + phi)*sin(n_ahrs3 + psi_) + cos(n_ahrs1 + phi)*cos(n_ahrs3 + psi_)*sin(n_ahrs2 + theta)) - y*(cos(n_ahrs1 + phi)*sin(n_ahrs3 + psi_) - cos(n_ahrs3 + psi_)*sin(n_ahrs1 + phi)*sin(n_ahrs2 + theta)) + x*cos(n_ahrs3 + psi_)*cos(n_ahrs2 + theta)), dT*cos(n_ahrs2 + theta)*sin(n_ahrs3 + psi_),  dT*(cos(n_ahrs1 + phi)*cos(n_ahrs3 + psi_) + sin(n_ahrs1 + phi)*sin(n_ahrs3 + psi_)*sin(n_ahrs2 + theta)), -dT*(cos(n_ahrs3 + psi_)*sin(n_ahrs1 + phi) - cos(n_ahrs1 + phi)*sin(n_ahrs3 + psi_)*sin(n_ahrs2 + theta));
                                                                                                                                    dT*(y*cos(n_ahrs1 + phi)*cos(n_ahrs2 + theta) - z*cos(n_ahrs2 + theta)*sin(n_ahrs1 + phi)),                                                            -dT*(x*cos(n_ahrs2 + theta) + z*cos(n_ahrs1 + phi)*sin(n_ahrs2 + theta) + y*sin(n_ahrs1 + phi)*sin(n_ahrs2 + theta)),                                                                                                                                                                                                                                                                      0,                    -dT*sin(n_ahrs2 + theta),                                                                 dT*cos(n_ahrs2 + theta)*sin(n_ahrs1 + phi),                                                                 dT*cos(n_ahrs1 + phi)*cos(n_ahrs2 + theta)];

    %% EKF: Predizione

    hat  =  hat + dT * J * vel;        
    P =  P + Lk * Q * Lk';            

 
end

== matlab function modello_completo_simulink2019/Navigation1/z_EKF/Trigger & Init/Depth trigger/MATLAB Function ==
  data: count input; count output; dT output; depth input; sum input; pulse output; prev output
function [count, dT, pulse, prev] = fcn(count, depth, sum)

% La funzione si occupa di monitorare la misura del profondimetro,
% quando essa è modificata manda un impulso al blocco EKF e il tempo
% trascorso dalla precedente variazione

dT = 0;  

if nnz(round(10.^4*sum )/10.^4) == 0
    pulse = 0;
    count = count + 1;
else
    pulse = 1;
    dT = count * (1/200);
    count = 1;
end

prev = depth;

== matlab function modello_completo_simulink2019/Env. & Sensor Model1/AHRS SENSOR/    ==
  data: ni_1 input; ni_1_dot input; lin_acc output; ang_vel output; m output; ni_2 input; eta_2 input; eta_2_dot input
function [lin_acc, ang_vel, m] = IMU(ni_1, ni_1_dot, ni_2, eta_2, eta_2_dot)

% questa funzione, partendo dalle informazioni cinematiche dell' AUV
% restituisce in output delle misure di accelerazione, velocità angolare
% e campo magnetico locale


% definisco R^T
% R = Rz(psi)*Ry(theta)*Rx(phi);

% yaw = psi; pitch = theta; roll = phi;

phi = eta_2(1);
theta = eta_2(2);
psi = eta_2(3);

R = [cos(psi)*cos(theta) cos(psi)*sin(theta)*sin(phi)-sin(psi)*cos(phi) cos(psi)*sin(theta)*cos(phi)+sin(psi)*sin(phi);
     sin(psi)*cos(theta) sin(psi)*sin(theta)*sin(phi)+cos(psi)*cos(phi) sin(psi)*sin(theta)*cos(phi)-cos(psi)*sin(phi);
    -sin(theta) cos(theta)*sin(phi) cos(theta)*cos(phi)];

% Rx_phi = [1 0 0; 0 cos(phi) sin(phi); 0 -sin(phi) cos(phi)];
% Ry_theta = [cos(theta) 0 -sin(theta); 0 1 0; sin(theta) 0 cos(theta)];
% Rz_psi = [cos(psi) sin(psi) 0; -sin(psi) cos(psi) 0; 0 0 1];

% R = Rz_psi'*Ry_theta'*Rx_phi;

% Definisco la matrice Jacobiana
 
%J_2 = [1 sin(phi)*tan(theta) cos(phi)*tan(theta);
%       0 cos(phi) -sin(phi);
%       0 sin(phi)/cos(theta) cos(phi)/cos(theta)];
  
% accelerometro

g = [0 0 9.82]; % [m/s^2]
 
%lin_acc = J_1' * (eta_1_ddot - g);  
 
% eta_1_ddot = J_1 * ni_1_dot + J_1_dot * ni_1

dphi = eta_2_dot(1);
dtheta = eta_2_dot(2);
dpsi = eta_2_dot(3);


J_1_dot = [-dtheta*(sin(theta)*cos(psi)) - dpsi*(sin(psi)*cos(theta)), ...
           dphi*(sin(psi)*sin(phi) + cos(psi)*sin(theta)*cos(phi)) + dtheta*(cos(psi)*cos(theta)*sin(phi)) - dpsi*(cos(psi)*cos(phi) + sin(psi)*sin(theta)*sin(phi)), ... 
           dphi*(sin(psi)*cos(phi) - cos(psi)*sin(theta)*sin(phi)) + dtheta*(cos(psi)*cos(theta)*cos(phi)) + dpsi*(cos(psi)*sin(phi) - sin(psi)*sin(theta)*cos(phi)); ...
          -dtheta*(sin(theta)*sin(psi)) + dpsi*(cos(psi)*cos(theta)), ...
           dphi*(-cos(psi)*sin(phi) + sin(psi)*sin(theta)*cos(phi)) + dtheta*(sin(psi)*cos(theta)*sin(phi)) + dpsi*(-sin(psi)*cos(phi) + cos(psi)*sin(theta)*sin(phi)), ... 
          -dphi*(cos(psi)*cos(phi) + sin(psi)*sin(theta)*sin(phi)) + dtheta*(sin(psi)*cos(theta)*cos(phi)) + dpsi*(sin(psi)*sin(phi) + cos(psi)*sin(theta)*cos(phi)); ...
          -dtheta*(cos(theta)), ...
           dphi*(cos(theta)*cos(phi)) - dtheta*(sin(theta)*sin(phi)), ...
          -dphi*(cos(theta)*sin(phi)) - dtheta*(sin(theta)*cos(phi))];

% J_1 = R;      

eta_1_ddot = R * ni_1_dot + J_1_dot * ni_1;

lin_acc = R' * (eta_1_ddot - g');
 
 
 %  giroscopio
 
 % se mi fosse stata fornita la eta_2_dot (espressa in terna NED, globale) la
 % misura del giroscopio sarebbe stata:
 
 %ang_vel = inv(J_2) * eta_2_dot;
 
 %avendo a disposizione in ingresso l'accelerazione in terna Body, la
 %misura della velocità angolare sarà:
 
 ang_vel = ni_2;
 
 % magnetometro ( campo magnetico terrestre espresso in terna NED)
 
 
% gaussian =  normrnd([0 0 0], [0.00131, 0.00094, 0.00157]);
% gaussian = incertezza dell'intensità del campo magnetico 
% calcolata su: https://www.ngdc.noaa.gov/geomag/calculators/magcalc.shtml#igrfwmm

 m_e = [0.238836 -0.010851 0.392423]'; % + gaussian';
 
 m = R' * m_e;
 
end

== matlab function modello_completo_simulink2019/Vehicle Model/Tau2T ==
  data: tau_des input; T output
function T= fcn(tau_des)
p1 = [0 -0.25 0]';
p2 = [0 0.25 0]';
p3 = [-0.25 0 0]';
p4 = [0.25 0 0]';
p5 = [-0.15 -0.15 0]';
p6 = [-0.15 0.15 0]';
p7 = [0.15 0 0]';

t1 = [1 0 0]';
t2 = t1;
t3 = [0 1 0]';
t4 = -t3;
t5 = [0 0 1]';
t6 = t5;
t7 = t5;

B1 = [t1; cross(p1,t1)];
B2 = [t2; cross(p2,t2)];
B3 = [t3; cross(p3,t3)];
B4 = [t4; cross(p4,t4)];
B5 = [t5; cross(p5,t5)];
B6 = [t6; cross(p6,t6)];
B7 = [t7; cross(p7,t7)];
B = [B1 B2 B3 B4 B5 B6 B7];

Bpinv=pinv(B);
T = Bpinv*tau_des;

end

== matlab function modello_completo_simulink2019/Navigation1/z_EKF/Trigger & Init/Initialization/MATLAB Function1 ==
  data: init_counter output; init_counter input; depth input; gps input; GPS_flag input; pulse output; init output; P0 output; prev output; diff_ input; store_gps input; gps_store output; store_depth input; depth_store output; num_cycle parameter
function [init_counter, pulse, init, P0, prev, gps_store, depth_store] = fcn_init(init_counter, depth, gps, GPS_flag, diff_, store_gps, store_depth, num_cycle)

% La funzione si occupa di valutare i valori iniziali dello stato e della varianza dell'errore di stima

%% Variabili
pulse = 0;
gps_store = store_gps;
depth_store = store_depth;
init = zeros(3,1);
P0 = zeros(3);
coder.extrinsic('init_position');

%%
if nnz(round(10.^4*diff_)/10.^4) ~= 0 && init_counter < num_cycle && GPS_flag == 1
    
    init_counter = init_counter + 1;
    gps_store(1, init_counter) = gps(1);
    gps_store(2, init_counter) = gps(2);
    pulse = 0;
    depth_store(init_counter) = depth;

        
elseif init_counter < num_cycle

    init_counter = init_counter;
    pulse = 0;
    
    
elseif init_counter >= num_cycle && init_counter < 300
   
    [init, P0] = init_position(store_gps, store_depth, num_cycle); 
    pulse = 1;
    init_counter = init_counter + 1;

else 
    
    pulse = 1;
   
end

prev = gps;

== matlab function modello_completo_simulink2019/Env. & Sensor Model1/DVL SENSOR/MATLAB Function ==
  data: ni input; niDVL output; c parameter
function niDVL = traslation(ni, c)
%Calcola la velocità in terna DVL

S = [0,-ni(6),ni(5); 
    ni(6),0,-ni(4); 
    -ni(5),ni(4),0];
p = [0;0;c];
niDVL = ni(1:3,1)+S*p;        %Formula fondamentale della cinematica

== matlab function modello_completo_simulink2019/Controller/AVVICINAMENTO/J2_inv ==
  data: tau_roll input; tau_or_body output; tau_pitch input; tau_yaw input; est_state input
function tau_or_body = fcn(tau_roll,tau_pitch,tau_yaw,est_state)
theta=est_state(1);
phi=est_state(2);
tau_or=[tau_roll;tau_pitch;tau_yaw];
J2_inv = [1       0          -sin(theta); 
         0   cos(phi)  cos(theta)*sin(phi);
         0  -sin(phi)  cos(theta)*cos(phi)];
tau_or_body=J2_inv*tau_or;
end

== matlab function modello_completo_simulink2019/Controller/GEODETIC2NED2/GEODETIC2NED1/MATLAB Function ==
  data: lat input; pos_s_Ned output; lon input
function pos_s_Ned = fcn(lat,lon)
coder.extrinsic('wgs84Ellipsoid','geodetic2ned');
pylonCenter = [43.723046;10.396635];
initPoint = [ 43.722984;10.396204;0];
hOrigin=0;
pos_s_Ned=zeros(3,1);
wgs84=wgs84Ellipsoid('meter');
lat0=pylonCenter(1);
lon0=pylonCenter(2);
h=initPoint(3);
h0=hOrigin;
[xs_N,ys_E,zs_D]=geodetic2ned(lat,lon,h,lat0,lon0,h0,wgs84);
pos_s_Ned=[xs_N,ys_E,zs_D]';
end

== matlab function modello_completo_simulink2019/Controller/GEODETIC2NED3/GEODETIC2NED/MATLAB Function ==
  data: lat input; lon input; pos_Ned output
function pos_Ned = fcn (lat,lon)
coder.extrinsic('wgs84Ellipsoid','geodetic2ned');
pylonCenter = [43.723046;10.396635];
initPoint = [ 43.722984;10.396204;0];
hOrigin=0;
pos_Ned=zeros(3,1);
wgs84=wgs84Ellipsoid('meter');
h=initPoint(3);
lat0=pylonCenter(1);
lon0=pylonCenter(2);
h0=hOrigin;
[x_N,y_E,z_D]=geodetic2ned(lat,lon,h,lat0,lon0,h0,wgs84);
pos_Ned=[x_N,y_E,z_D]';
end

== matlab function modello_completo_simulink2019/Controller/IMMERSIONE//RISALITA/J2_inv ==
  data: tau_roll input; tau_or_body output; tau_pitch input; tau_yaw input; est_state input
function tau_or_body = fcn(tau_roll,tau_pitch,tau_yaw,est_state)
theta=est_state(1);
phi=est_state(2);
tau_or=[tau_roll;tau_pitch;tau_yaw];
J2_inv = [1       0          -sin(theta); 
         0   cos(phi)  cos(theta)*sin(phi);
         0  -sin(phi)  cos(theta)*cos(phi)];
tau_or_body=J2_inv*tau_or;
end

== matlab function modello_completo_simulink2019/Env. & Sensor Model1/Sonar sensor/MATLAB Function ==
  data: xNorth input; s output; yEast input; zDown input; roll input; pitch input; yaw input; pylonRadius parameter; s_data parameter; son output
function [s,son] = Sonar_ideal(xNorth,yEast,zDown,roll,pitch,yaw,pylonRadius, s_data)

coder.extrinsic('Sonar_id');

s_data.num = 5;
s = zeros(s_data.num,1);
son = zeros(s_data.num,5);

[s,son] = Sonar_id(xNorth,yEast,zDown,roll,pitch,yaw,pylonRadius,s_data);

== matlab function modello_completo_simulink2019/Controller/MATLAB Function1 ==
  data: STATE input; EN output; bodyposx_err input; yaw_err input; depth_err input; INSP input string
function EN = fcn(STATE,bodyposx_err,yaw_err,depth_err, INSP)

%EN(1)= bodypos_err
%EN(2)= rel_dist_err
%EN(3)=surge_err
%EN(4)= latvel_err
%EN(5)=depth_err
%EN(6)= RP_err
%EN(7)= rel_or_err
%EN(8)= yaw_err

EN=zeros(1,8)';

if (STATE == 101)
    EN(8)=1;
end
%avvicinamento pilone
if (STATE== 102)
    EN(8)=1;
    EN(3)=1;
    if (STATE==102) && (bodyposx_err<=3)
        EN(8)=1;
        EN(1)=1;
        EN(3)=0;
    end
end
%rotazione attorno al pilone in superficie
if (STATE == 103)
    EN(2)=1;
    EN(7)=1;
    EN(4)=1;    
    if (yaw_err<=10)
        EN(4)=0;
        EN(8)=1;
        EN(2)=1;
        EN(7)=0;
    end
end
%unicodestr = native2unicode(INSP);
s1=INSP;
s2='vertical';
CMP=strcmp(s1,s2);
if (CMP == 1) %inizio ispezione verticale
    if (STATE==201) 
        EN(2)=1;
        EN(5)=1;
        EN(7)=1;
        EN(6)=1;
        if(depth_err<=3) %stacco i thrusters che controllano la depth
            EN(2)=1;
            EN(7)=1;
            EN(5)=0;
            EN(6)=1;   
        end
    end
    if(STATE==202) && (depth_err<0.2) %controllo di velocità laterale
        EN(2)=1;
        EN(4)=1;
        EN(5)=1;
        EN(6)=1;
        EN(7)=1;
        if(yaw_err<=10) %switch su controllo di posizione
            EN(8)=1;
            EN(2)=1;
            EN(7)=0;
            EN(4)=0; 
            EN(5)=1;
            EN(6)=1;
        end
    end  %fine ispezione verticale
else
    if (STATE==202) && (depth_err<0.2) % inizio ispezione orizzontale
        EN(2)=1;
        EN(5)=1;
        EN(4)=1;  
        EN(7)=1;  
        EN(6)=1;
        if(yaw_err<=10) %switch su controllo di yaw
            EN(8)=1;
            EN(2)=1;
            EN(7)=0; 
            EN(4)=0;
            EN(5)=1;
            EN(6)=1;
        end
    end
    if (STATE==201) %transetto verticale in isp. orizzontale
        EN(2)=1;
        EN(7)=1;
        EN(5)=1;
        EN(6)=1;   
    end 
end     %fine ispezione orizzontale
%fase di immersione   
if(STATE==104)
   EN(2)=1;
   EN(7)=1;
   EN(5)=1;
   EN(6)=1;
   if(depth_err<=3) %stacco i thrusters che controllano la depth
        EN(2)=1;
        EN(7)=1;
        EN(5)=0;
        EN(6)=1;   
   end
end
%fase di risalita
if(STATE==401)
   EN(2)=1;
   EN(7)=1;
   EN(5)=1;
   EN(6)=1;
end   
   
%fase di errore e fine missione
if(STATE == 500) || (STATE == 999)% lascio così poichè in caso di errore
   EN=zeros(1,8)';               % comunque spegnamo tutti i segnali e
                                % lo facciamo risalire attraverso i 4N
end
end

== matlab function modello_completo_simulink2019/Controller/NED2BODY ==
  data: eta1_dot input; mi1 output; phi input; theta input; psi input
function mi1 = fcn(eta1_dot,phi,theta,psi)
Rx_phi=[1 0 0;0 cos(phi) -sin(phi);0 sin(phi) cos(phi)];
Ry_theta=[cos(theta) 0 sin(theta);0 1 0;-sin(theta) 0 cos(theta)];
Rz_psi=[cos(psi) -sin(psi) 0;sin(psi) cos(psi) 0;0 0 1];
J1=Rx_phi*Ry_theta*Rz_psi;
mi1 =J1^-1*eta1_dot;

== matlab function modello_completo_simulink2019/Controller/NED2BODY1 ==
  data: abspos_err input; bodypos_err output; phi input; theta input; psi input
function bodypos_err = fcn(abspos_err,phi,theta,psi)
Rx_phi=   [1      0        0;
           0   cos(phi) -sin(phi);
           0   sin(phi) cos(phi)];
    
Ry_theta=[cos(theta) 0  sin(theta);
              0      1      0;
         -sin(theta) 0  cos(theta)];
     
Rz_psi=  [cos(psi) -sin(psi)  0;
          sin(psi)  cos(psi)  0;
           0           0      1];
       
J1=Rx_phi*Ry_theta*Rz_psi;
bodypos_err=J1^-1*abspos_err;

== matlab function modello_completo_simulink2019/Controller/POSIZIONAMENTO/J2_inv ==
  data: tau_roll input; tau_or_body output; tau_pitch input; tau_yaw input; est_state input
function tau_or_body = fcn(tau_roll,tau_pitch,tau_yaw,est_state)
theta=est_state(1);
phi=est_state(2);
tau_or=[tau_roll;tau_pitch;tau_yaw];
J2_inv = [1       0          -sin(theta); 
         0   cos(phi)  cos(theta)*sin(phi);
         0  -sin(phi)  cos(theta)*cos(phi)];
tau_or_body=J2_inv*tau_or;
end

== matlab function modello_completo_simulink2019/Controller/ROTAZIONE IN PROFONDITA'/J2_inv ==
  data: tau_roll input; tau_or_body output; tau_pitch input; tau_yaw input; est_state input
function tau_or_body = fcn(tau_roll,tau_pitch,tau_yaw,est_state)
theta=est_state(1);
phi=est_state(2);
tau_or=[tau_roll;tau_pitch;tau_yaw];
J2_inv = [1       0          -sin(theta); 
         0   cos(phi)  cos(theta)*sin(phi);
         0  -sin(phi)  cos(theta)*cos(phi)];
tau_or_body=J2_inv*tau_or;
end

== matlab function modello_completo_simulink2019/Controller/ROTAZIONE IN SUPERFICIE/J2_inv ==
  data: tau_roll input; tau_or_body output; tau_pitch input; tau_yaw input; est_state input
function tau_or_body = fcn(tau_roll,tau_pitch,tau_yaw,est_state)
theta=est_state(1);
phi=est_state(2);
tau_or=[tau_roll;tau_pitch;tau_yaw];
J2_inv = [1       0          -sin(theta); 
         0   cos(phi)  cos(theta)*sin(phi);
         0  -sin(phi)  cos(theta)*cos(phi)];
tau_or_body=J2_inv*tau_or;
end

== matlab function modello_completo_simulink2019/Controller/T2n/MATLAB Function ==
  data: Tdes input; n output
function n  = fcn(Tdes)
n=zeros(1,7)';
a1=0.000388302366464000;
%assunzione modello a bassa velocità
for i=1:1:7
       n(i)=sign(Tdes(i))*sqrt((abs(Tdes(i))/a1));  
end
end

== matlab function modello_completo_simulink2019/Controller/Tau2T/Tau2T ==
  data: tau_des input; T output
function T= fcn(tau_des)
p1 = [0 -0.25 0]';
p2 = [0 0.25 0]';
p3 = [-0.25 0 0]';
p4 = [0.25 0 0]';
p5 = [-0.15 -0.15 0]';
p6 = [-0.15 0.15 0]';
p7 = [0.15 0 0]';

t1 = [1 0 0]';
t2 = t1;
t3 = [0 1 0]';
t4 = -t3;
t5 = [0 0 1]';
t6 = t5;
t7 = t5;

B1 = [t1; cross(p1,t1)];
B2 = [t2; cross(p2,t2)];
B3 = [t3; cross(p3,t3)];
B4 = [t4; cross(p4,t4)];
B5 = [t5; cross(p5,t5)];
B6 = [t6; cross(p6,t6)];
B7 = [t7; cross(p7,t7)];
B = [B1 B2 B3 B4 B5 B6 B7];

Bpinv=pinv(B);
T = Bpinv*tau_des;

end

== matlab function modello_completo_simulink2019/Controller/Tau2T/Tau_des ENABLE ==
  data: STATE input; tau_des output; tau1 input; tau2 input; tau3 input; tau4 input; tau5 input
function tau_des= fcn(STATE,tau1,tau2,tau3,tau4,tau5)
tau_des= zeros(1,6)';
if (STATE==101)
    tau_des=tau1;
end
if (STATE==102)
    tau_des=tau2;
end
if (STATE==103)
    tau_des= tau3;
end
if (STATE== 201|| STATE==104||STATE==401)
    tau_des=tau4;
end
if (STATE== 202)
    tau_des=tau5;
end
if (STATE==500 || STATE== 999)
    tau_des=zeros(1,6)';
end
end

== matlab function modello_completo_simulink2019/Controller/wrapTopi ==
  data: u input; y output
function y = fcn(u)
coder.extrinsic('wrapToPi');
y=0;
y = wrapToPi(u);
end
